simulink model "ysw13_5"  (Simulink 8.3)
settings: Solver=ode4  StartTime=0.0  StopTime=2  RelTol=1e-3
settings Model: Creator=Administrator  LastModifiedBy=Administrator  ExtModeTrigMode=oneshot  ExtModeArmWhenConnect=off
settings DataIOCC: Decimation=100  LimitDataPoints=off  SaveOutput=off  SaveTime=off
settings OptimizationCC: BlockReduction=off  BooleanDataType=off  InitFltsAndDblsToZero=on
settings DebuggingCC: SaveWithParameterizedLinksMsg=none  SignalResolutionControl=TryResolveAllWithWarning  SolverPrmCheckMsg=none  MultiTaskDSMMsg=warning  MultiTaskCondExecSysMsg=none  FcnCallInpInsideContextMsg=UseLocalSettings  StateNameClashWarn=none
settings HardwareCC: TargetUnknown=on
settings RTWCC: IncludeERTFirstTime=on
settings GRTTargetCC: TargetFcnLib=ansi_tfl_tmw.mat

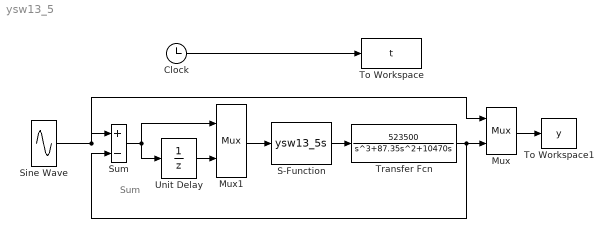
== system ysw13_5 ==
  note: Sum
  Clock : Clock
  Mux : Mux  Inputs=2
  Mux1 : Mux  Inputs=2
  S-Function : S-Function  FunctionName=ysw13_5s  EnableBusSupport=off
  Sine Wave : Sin  Frequency=1*2*pi  SampleTime=0.001
  Sum : Sum  Inputs=|+-  SaturateOnIntegerOverflow=on  InputSameDT=on  OutDataTypeStr=Inherit: Same as first input
  To Workspace : ToWorkspace  VariableName=t  SampleTime=-1
  To Workspace1 : ToWorkspace  VariableName=y  SampleTime=-1
  Transfer Fcn : TransferFcn  Numerator=[523500]  Denominator=[1 87.35 10470 0]
  Unit Delay : UnitDelay  SampleTime=0.001
  wires:
  Sine Wave/1 -> Sum/1, Mux/1
  Mux1/1 -> S-Function/1
  Unit Delay/1 -> Mux1/2
  Sum/1 -> Mux1/1, Unit Delay/1
  S-Function/1 -> Transfer Fcn/1
  Mux/1 -> To Workspace1/1
  Transfer Fcn/1 -> Mux/2, Sum/2
  Clock/1 -> To Workspace/1
